simulink model "overrun"  (Simulink 4.00)
settings: Solver=ode45  StartTime=0.0  StopTime=2  RelTol=1e-3
InitFcn:
  | clear functions
libraries: truetime x1
settings Model: Creator=anton  LastModifiedBy=anton  OutputTimes=[0.00199]  SaveTime=off  SaveOutput=off  LimitDataPoints=off  ExtModeTrigMode=oneshot  ExtModeArmWhenConnect=off  ExtModeAutoUpdateStatusClock=off  BlockReductionOpt=off

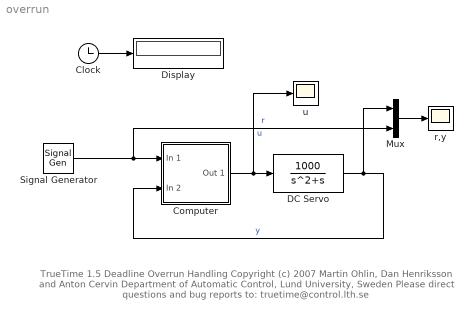
== system overrun ==
  note: TrueTime 1.5  Deadline Overrun Handling
      | Copyright (c) 2007
      | Martin Ohlin, Dan Henriksson and Anton Cervin
      | Department of Automatic Control, Lund University, Sweden
      | Please direct questions and bug reports to:  truetime@control.lth.se
  Clock : Clock
      settings: DisplayTime=off  Decimation=10
  Computer : Subsystem
      settings: RTWFcnNameOpts=Auto  RTWFileNameOpts=Auto
  DC Servo : TransferFcn  Numerator=[1000]  Denominator=[1 1 0]  AbsoluteTolerance=auto  Realization=auto
  Display : Display
      settings: Format=short
  Mux : Mux  Inputs=2
  Signal Generator : SignalGenerator  WaveForm=square  Amplitude=0.75  Frequency=1.5  Units=Hertz
  r,y : Scope
      settings: TimeRange=2  YMin=-1.5  YMax=1.5  SaveToWorkspace=off  SaveName=ScopeData  MaxDataPoints=120000
  u : Scope
      settings: TimeRange=2  YMin=-1.5  YMax=1.5  SaveToWorkspace=off  MaxDataPoints=120000
  wires:
  Computer/1(Out 1) -> DC Servo/1, u/1  "u"
  Mux/1 -> r,y/1
  Signal Generator/1 -> Computer/1(In 1), Mux/2  "r"
  Clock/1 -> Display/1
  DC Servo/1 -> Computer/2(In 2), Mux/1  "y"

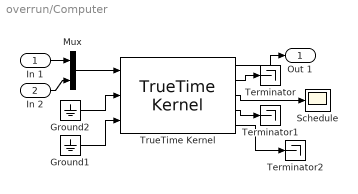
== system overrun/Computer ==
  In 1 : Inport  Port=1  LatchInput=off
  In 2 : Inport  Port=2  LatchInput=off
  Ground1 : Ground
  Ground2 : Ground
  Mux : Mux  Inputs=2
  Schedule : Scope
      settings: TickLabels=on  TimeRange=2  YMin=0.8  YMax=1.7  SaveToWorkspace=off  SaveName=ScopeData  DataFormat=Array  MaxDataPoints=5000
  Terminator : Terminator
  Terminator1 : Terminator
  Terminator2 : Terminator
  TrueTime Kernel : truetime/TrueTime Kernel  sfun=overrun_init  args=0  battery=off  clockdrift=0  clockoffset=0
  Out 1 : Outport  Port=1
  wires:
  In 1/1 -> Mux/1
  TrueTime Kernel/1 -> Out 1/1
  TrueTime Kernel/2 -> Terminator/1
  TrueTime Kernel/4 -> Terminator1/1
  TrueTime Kernel/3 -> Schedule/1
  Ground2/1 -> TrueTime Kernel/2
  Ground1/1 -> TrueTime Kernel/3
  Mux/1 -> TrueTime Kernel/1
  In 2/1 -> Mux/2
  TrueTime Kernel/5 -> Terminator2/1
